simulink model "test1"  (R2022b)
settings: Solver=ode4  StartTime=0.0  StopTime=100  FixedStep=0.1  RelTol=1e-3
settings Model: Creator=a1pab  LastModifiedBy=a1pab

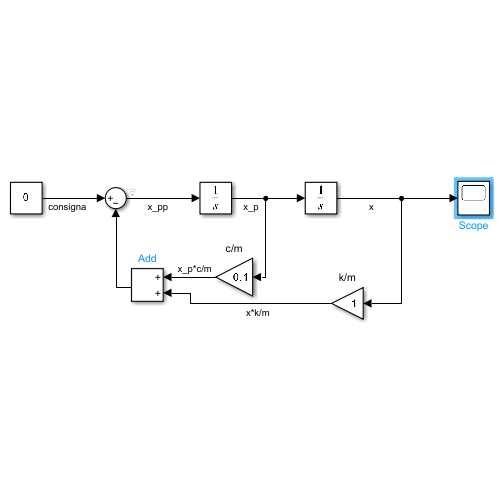
[thumbnail: Simulink's stored preview of the top-level diagram]
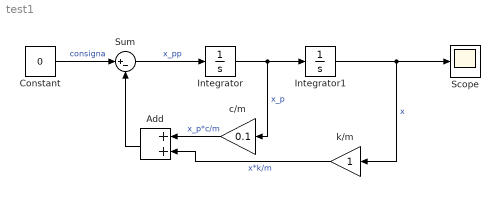
== system test1 ==
  Add : Sum
  Constant : Constant  Value=0
  Integrator : Integrator
  Integrator1 : Integrator  InitialCondition=1
  Scope : Scope
  Sum : Sum  Inputs=|+-
  c/m : Gain  Gain=0.1
  k/m : Gain
  wires:
  Sum/1 -> Integrator/1  "x_pp"
  Integrator/1 -> c/m/1, Integrator1/1  "x_p"
  Integrator1/1 -> Scope/1, k/m/1  "x"
  k/m/1 -> Add/2  "x*k/m"
  Constant/1 -> Sum/1  "consigna"
  Add/1 -> Sum/2
  c/m/1 -> Add/1  "x_p*c/m"
